simulink model "CT_simpletaskfunctionWithgain_02"  (R2015a)
settings: Solver=ode45  StartTime=0.0  StopTime=10.0  RelTol=1e-3
libraries: simulink x1
settings Model: Creator=Abu Bakar  LastModifiedBy=Abu Bakar

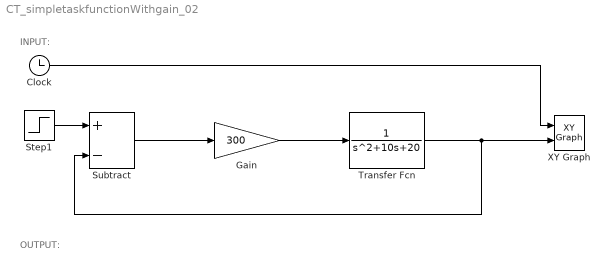
== system CT_simpletaskfunctionWithgain_02 ==
  note: OUTPUT:
  note: INPUT:
  Clock : Clock
  Gain : Gain  Gain=300  OutMin=[300]  OutMax=[300]
  Step1 : Step  Time=0.06  SampleTime=0
  Subtract : Sum  Inputs=+-
  Transfer Fcn : TransferFcn  Denominator=[1 10 20]
  XY Graph : simulink/Sinks/XY Graph  xmin=0  xmax=10  ymin=-1  ymax=5  st=-1
  wires:
  Transfer Fcn/1 -> XY Graph/2, Subtract/2
  Clock/1 -> XY Graph/1
  Step1/1 -> Subtract/1
  Subtract/1 -> Gain/1
  Gain/1 -> Transfer Fcn/1
